simulink model "Discrete_Time_either_ic_verif"  (Simulink 8.4)
settings: Solver=ode45  StartTime=0.0  StopTime=10.0  RelTol=1e-3
undefined symbols (not defined in the file): DiscIntNeverNeededParam, sigbuilder_block
settings Model: Creator=Romain  LastModifiedBy=hbourbou
settings DataIOCC: SignalLoggingSaveFormat=Dataset
settings OptimizationCC: ExpressionDepthLimit=128
settings DebuggingCC: SolverPrmCheckMsg=none  FcnCallInpInsideContextMsg=EnableAllAsError  FrameProcessingCompatibilityMsg=error  StateNameClashWarn=none
settings GRTTargetCC: CombineOutputUpdateFcns=on  GRTInterface=off

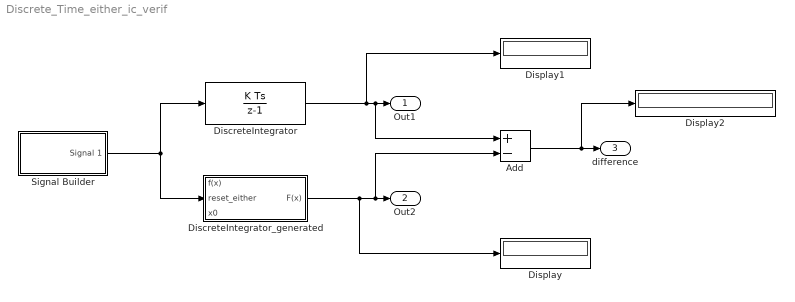
== system Discrete_Time_either_ic_verif ==
  Add : Sum  Inputs=+-
  DiscreteIntegrator : DiscreteIntegrator  ExternalReset=either  InitialConditionSource=external  InitialConditionSetting=State (most efficient)  SampleTime=-1  ICPrevOutput=DiscIntNeverNeededParam  ICPrevScaledInput=DiscIntNeverNeededParam
  DiscreteIntegrator_generated : Subsystem  TreatAsAtomicUnit=on
  Display : Display
  Display1 : Display
  Display2 : Display
  Signal Builder : Subsystem  Tag=STV Subsys  LoadFcn=sigbuilder_block('load');  StartFcn=sigbuilder_block('start');  StopFcn=sigbuilder_block('stop');  ClipboardFcn=sigbuilder_block('clipboard');  mask(Sigbuilder block){}
      mask help: Simulink:masks:SigbuilderBlock_MD
      mask init:
      | if ~strcmp(get_param(bdroot(gcbh),'SimulationStatus'),'stopped') tuvar = sigbuilder_block('maskInit'); end
      settings: CopyFcn=sigbuilder_block('copy');  DeleteFcn=sigbuilder_block('delete');  ModelCloseFcn=sigbuilder_block('modelClose');  PreSaveFcn=sigbuilder_block('preSave');  PauseFcn=sigbuilder_block('pause');  ContinueFcn=sigbuilder_block('continue');  NameChangeFcn=sigbuilder_block('namechange');  OpenFcn=sigbuilder_block('open',[437.6 199.2 550.4 400 ]);  CloseFcn=sigbuilder_block('close');
      mask Display: plot(0, 0, 100, 100,[2, 2, 32, 32, 2], [68, 8, 8, 68, 68],[32, 2], [38, 38], [32, 19, 2],[53, 60, 44], [32, 17, 17, 2],[16, 16, 31, 31]);txt = getActiveGroup(gcbh);text(2, 100, txt,'verticalAlignment', 'top');
  Out1 : Outport
  Out2 : Outport  Port=2
  difference : Outport  Port=3
  wires:
  Signal Builder/1(Signal 1) -> DiscreteIntegrator_generated/2(reset_either), DiscreteIntegrator/2
  DiscreteIntegrator/1 -> Display1/1, Add/1, Out1/1
  DiscreteIntegrator_generated/1(F(x)) -> Display/1, Add/2, Out2/1
  Add/1 -> Display2/1, difference/1

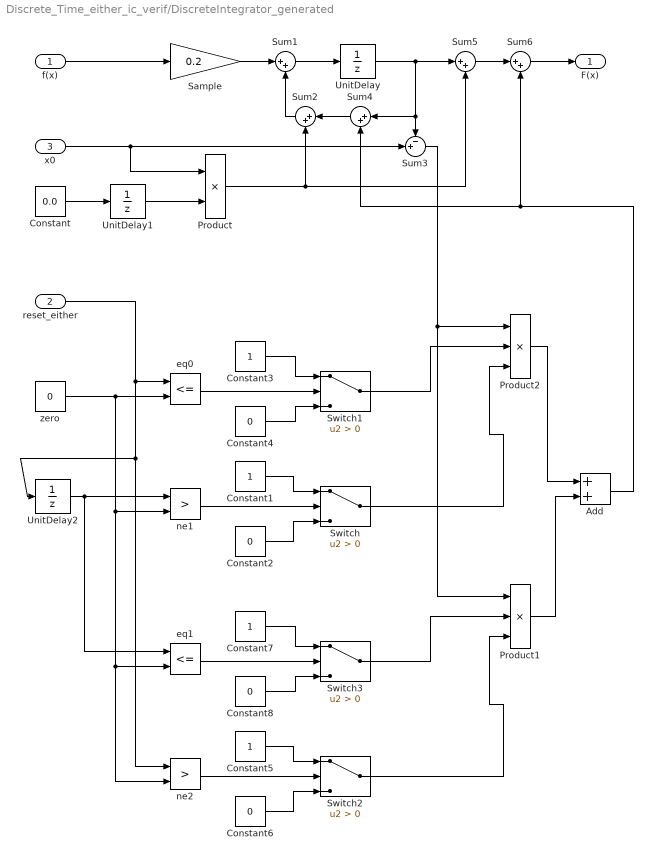
== system Discrete_Time_either_ic_verif/DiscreteIntegrator_generated ==
  f(x) : Inport
  reset_either : Inport  Port=2
  x0 : Inport  Port=3
  Add : Sum
  Constant : Constant  Value=0.0  SampleTime=-1
  Constant{1,3,5,7} (4 alike) : Constant
  Constant{2,4,6,8} (4 alike) : Constant  Value=0
  Product : Product  RndMeth=Zero
  Product1 : Product  Inputs=3  RndMeth=Zero
  Product2 : Product  Inputs=3  RndMeth=Zero
  Sample : Gain  Gain=0.2
  Sum1 : Sum  RequirementInfo={} %GIDa_f96f33ca_03e6_4638_9d3f_e25ea3bec852  Inputs=|++
  Sum2 : Sum  RequirementInfo={} %GIDa_cfda0997_5afc_4b05_b848_2fcebfcc0a97  Inputs=|++
  Sum3 : Sum  RequirementInfo={} %GIDa_d7168430_20b9_4ab3_9b80_5feadc14d142  Inputs=-+|
  Sum4 : Sum  RequirementInfo={} %GIDa_8fb3df74_f003_445d_8a46_b2d778a1e3c3  Inputs=|++
  Sum5 : Sum  RequirementInfo={} %GIDa_2b04bd8f_9136_4794_bc70_bd35290710f7  Inputs=|++
  Sum6 : Sum  RequirementInfo={} %GIDa_a1136b78_9cda_458c_adae_d5f2d8fb27cd  Inputs=|++  SampleTime=0.2
  Switch{,1..3} (4 alike) : Switch  Criteria=u2 > Threshold
  UnitDelay : UnitDelay  SampleTime=0.2
  UnitDelay1 : UnitDelay  InitialCondition=1  SampleTime=0.2
  UnitDelay2 : UnitDelay  SampleTime=0.2
  eq0 : RelationalOperator  Operator=<=  OutDataTypeStr=boolean
  eq1 : RelationalOperator  Operator=<=  OutDataTypeStr=boolean
  ne1 : RelationalOperator  Operator=>  OutDataTypeStr=boolean
  ne2 : RelationalOperator  Operator=>  OutDataTypeStr=boolean
  zero : Constant  Value=0  SampleTime=-1
  F(x) : Outport  RequirementInfo={} %GIDa_ab7433f0_031f_481c_bcc3_779a828b4a51
  wires:
  Sum1/1 -> UnitDelay/1
  Sample/1 -> Sum1/1
  UnitDelay/1 -> Sum5/1, Sum3/1, Sum4/1
  Sum2/1 -> Sum1/2
  Product/1 -> Sum5/2, Sum2/2
  UnitDelay1/1 -> Product/2
  Constant/1 -> UnitDelay1/1
  x0/1 -> Product/1, Sum3/2
  Sum4/1 -> Sum2/1
  Add/1 -> Sum6/2, Sum4/2
  f(x)/1 -> Sample/1
  Sum5/1 -> Sum6/1
  Sum6/1 -> F(x)/1
  ne1/1 -> Switch/2
  Constant1/1 -> Switch/1
  Constant2/1 -> Switch/3
  Switch/1 -> Product2/3
  eq0/1 -> Switch1/2
  Constant3/1 -> Switch1/1
  Constant4/1 -> Switch1/3
  Switch1/1 -> Product2/2
  UnitDelay2/1 -> eq1/1, ne1/1
  reset_either/1 -> ne2/1, UnitDelay2/1, eq0/1
  Sum3/1 -> Product1/1, Product2/1
  zero/1 -> ne2/2, eq1/2, ne1/2, eq0/2
  ne2/1 -> Switch2/2
  Constant5/1 -> Switch2/1
  Constant6/1 -> Switch2/3
  Switch2/1 -> Product1/3
  eq1/1 -> Switch3/2
  Constant7/1 -> Switch3/1
  Constant8/1 -> Switch3/3
  Switch3/1 -> Product1/2
  Product1/1 -> Add/2
  Product2/1 -> Add/1

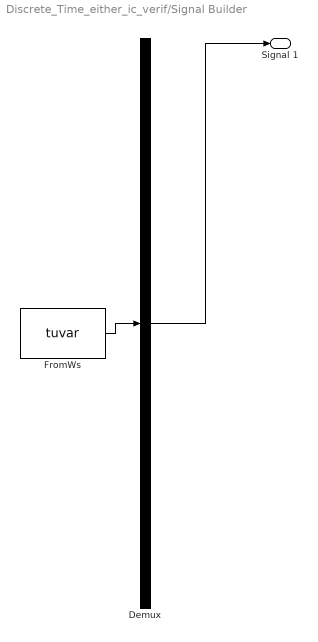
== system Discrete_Time_either_ic_verif/Signal Builder ==
  Demux : Demux  Tag=STV Demux  Outputs=1
  FromWs : FromWorkspace  Tag=STV FromWs  VariableName=tuvar  SampleTime=0  SigBuilderData=DataTag0  VnvData=DataTag1
      SigBuilderData=|
      | common.afterFinalStr = 'Extrapolate'
      | common.sampleTime = 0
      | dataSet.timeRange = [0 10]
      | dataSet.name = 'Group 1'
      | sbobj.Groups.Name = 'Group 1'
      | sbobj.Groups.Signals.Name = 'Signal 1'
      | sbobj.Groups.Signals.XData = [0 4 4 6 6 10]
      | sbobj.Groups.Signals.YData = [0 0.99 1 0.3 0.26 0]
  Signal 1 : Outport  Tag=STV Outport
  wires:
  Demux/1 -> Signal 1/1
  FromWs/1 -> Demux/1
